simulink model "Assignment_1_3K04"  (R2022b)
settings: Solver=FixedStepAuto  StartTime=0.0  StopTime=1  FixedStep=1e-3  RelTol=1e-3  EnableMultiTasking=on
undefined symbols (not defined in the file): D0, D1, D10, D11, D12, D13, D2, D3, D4, D5, D6, D7, D8, D9, PTA0, PTA1, PTA2, PTB23, PTB9, PTC16, PTC17, PTC2, PTC3, PTC4, PTD0, PTD1, PTD2, PTD3
libraries: frdmk64flib x14
settings Model: ExtModeTrigDuration=5  Creator=Stephen Oh  LastModifiedBy=rebec
settings SolverCC: AlgebraicLoopSolver=TrustRegion
settings OptimizationCC: EnhancedBackFolding=on  PassReuseOutputArgsAs=Individual arguments  ZeroExternalMemoryAtStartup=off  ZeroInternalMemoryAtStartup=off  MaxStackSize=64  OptimizeBlockOrder=speed  DifferentSizesBufferReuse=on  OptimizationCustomize=off  EfficientTunableParamExpr=on
settings DebuggingCC: ParameterTunabilityLossMsg=error  UnconnectedInputMsg=warning  UnconnectedOutputMsg=warning  UnconnectedLineMsg=warning  SFMachineParentedDataDiag=warning
settings HardwareCC: ProdBitPerPointer=32  ProdBitPerSizeT=32  ProdBitPerPtrDiffT=32  ProdLargestAtomicInteger=Long  ProdLargestAtomicFloat=Double  ProdWordSize=32  ProdHWDeviceType=ARM Compatible->ARM Cortex
settings ModelReferenceCC: EnableRefExpFcnMdlSchedulingChecks=on
settings SFSimCC: MATLABDynamicMemAlloc=off
settings RTWCC: Description=Embedded Coder  SystemTargetFile=ert.tlc  HardwareBoard=NXP FRDM-K64F  TLCOptions="-aInlineSetEventsForThisBaseRateFcn=TLC_FALSE -aSuppressMultiTaskScheduler=TLC_FALSE  -aRateBasedStepFcn=0"  TemplateMakefile=ert_default_tmf  Toolchain=GNU Tools for ARM Embedded Processors
settings CodeAppCC: ForceParamTrailComments=on  IgnoreCustomStorageClasses=off  OperatorAnnotations=on  SimulinkDataObjDesc=on  SFDataObjDesc=on  InsertBlockDesc=on

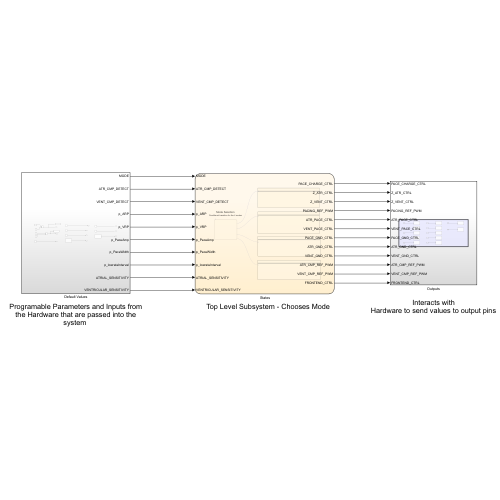
[thumbnail: Simulink's stored preview of the top-level diagram]
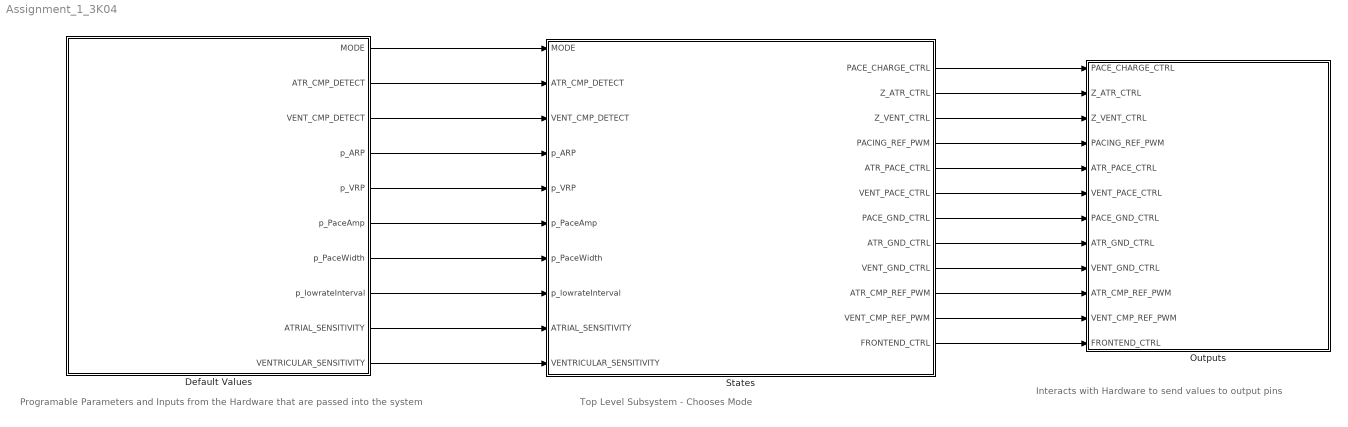
== system Assignment_1_3K04 ==
  note: Programable Parameters and Inputs from the Hardware that are passed into the system
  note: Top Level Subsystem - Chooses Mode
  note: Interacts with
      | Hardware to send values to output pins
  " States" : Stateflow chart  TreatAsAtomicUnit=on
      settings: PortSchema="{\"entries\":[{\"content\":{\"sides\":[{\"content\":{\"connectorIds\":[\"In1\",\"In2\",\"In3\",\"In4\",\"In5\",\"In6\",\"In7\",\"In8\",\"In9\",\"In10\"]},\"type\":\"ConnectorPlacement.EquallySpacedRectSide\",\"uuid\":\"15e03f69-5c25-4f3e-b3fb-d71978e552f4\"},{\"content\":{\"connectorIds\":[\"Out7\",\"Out4\",\"Out5\",\"Out8\",\"Out9\",\"Out3\",\"Out6\",\"Out1\",\"Out2\",\"Out10\",\"Out12\",\"Out11\"],\"side\":\"RIGHT\"},\"type\":\"ConnectorPlacement.EquallySpacedRectSide\",\"uuid\":\"02171bf1-edb1-4b01-9e56-a8642c556ed6\"},{\"content\":{\"connectorIds\":[],\"side\":\"TOP\"},\"type\":\"ConnectorPlacement.EquallySpacedRectSide\",\"uuid\":\"cc6b5506-3435-4740-9e3f-4dfe15d30bff\"}]},\"type\":\"ConnectorPlacement.EquallySpacedConnector\",\"uuid\":\"0ad55da7-1e65-48d0-a0a4-2620ffa94320\"}],\"packageUris\":[\"http://schema.mathworks.com/mf0/Connector/R2020b\"],\"version\":\"1.0\"}"
  Default Values : Subsystem
  Outputs : Subsystem
  wires:
  Default Values/1(MODE) -> " States"/1(MODE)
  Default Values/2(ATR_CMP_DETECT) -> " States"/2(ATR_CMP_DETECT)
  Default Values/3(VENT_CMP_DETECT) -> " States"/3(VENT_CMP_DETECT)
  Default Values/4(p_ARP) -> " States"/4(p_ARP)
  Default Values/5(p_VRP) -> " States"/5(p_VRP)
  Default Values/7(p_PaceWidth) -> " States"/7(p_PaceWidth)
  Default Values/9(ATRIAL_SENSITIVITY) -> " States"/9(ATRIAL_SENSITIVITY)
  Default Values/10(VENTRICULAR_SENSITIVITY) -> " States"/10(VENTRICULAR_SENSITIVITY)
  " States"/7(PACE_CHARGE_CTRL) -> Outputs/1(PACE_CHARGE_CTRL)
  " States"/4(Z_ATR_CTRL) -> Outputs/2(Z_ATR_CTRL)
  " States"/5(Z_VENT_CTRL) -> Outputs/3(Z_VENT_CTRL)
  " States"/8(PACING_REF_PWM) -> Outputs/4(PACING_REF_PWM)
  " States"/9(ATR_PACE_CTRL) -> Outputs/5(ATR_PACE_CTRL)
  " States"/3(VENT_PACE_CTRL) -> Outputs/6(VENT_PACE_CTRL)
  " States"/6(PACE_GND_CTRL) -> Outputs/7(PACE_GND_CTRL)
  " States"/1(ATR_GND_CTRL) -> Outputs/8(ATR_GND_CTRL)
  " States"/2(VENT_GND_CTRL) -> Outputs/9(VENT_GND_CTRL)
  " States"/10(ATR_CMP_REF_PWM) -> Outputs/10(ATR_CMP_REF_PWM)
  " States"/12(VENT_CMP_REF_PWM) -> Outputs/11(VENT_CMP_REF_PWM)
  " States"/11(FRONTEND_CTRL) -> Outputs/12(FRONTEND_CTRL)
  Default Values/8(p_lowrateInterval) -> " States"/8(p_lowrateInterval)
  Default Values/6(p_PaceAmp) -> " States"/6(p_PaceAmp)

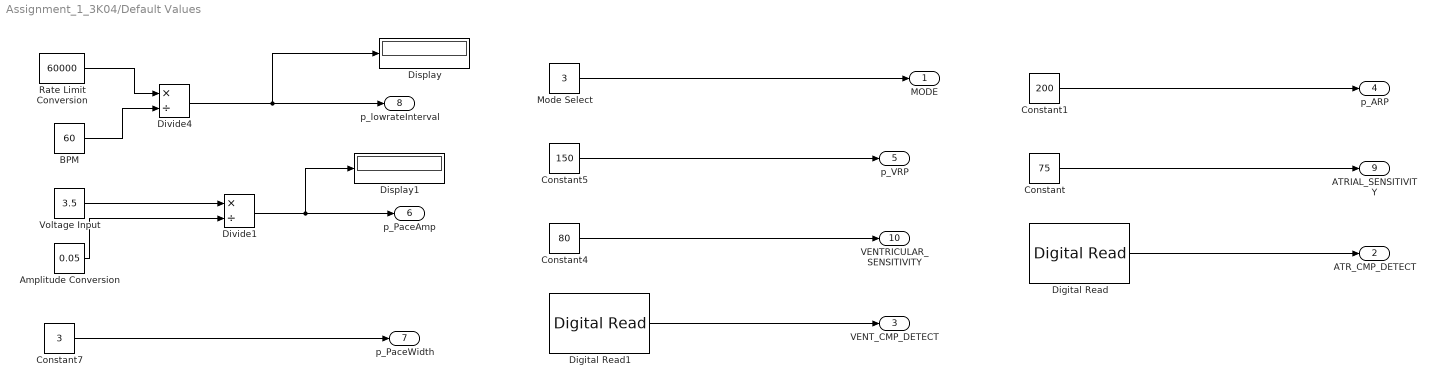
== system Assignment_1_3K04/Default Values ==
  Amplitude Conversion : Constant  Value=0.05
  BPM : Constant  Value=60
  Constant : Constant  Value=75
  Constant1 : Constant  Value=200
  Constant4 : Constant  Value=80
  Constant5 : Constant  Value=150
  Constant7 : Constant  Value=3
  Digital Read : frdmk64flib/Digital Read  Whichpin=PTC16 (D0)  SampleTime=-1
  Digital Read1 : frdmk64flib/Digital Read  Whichpin=PTC17 (D1)  SampleTime=-1
  Display : Display
  Display1 : Display
  Divide1 : Product  Inputs=*/  RndMeth=Nearest
  Divide4 : Product  Inputs=*/  OutDataTypeStr=Inherit: Keep MSB  RndMeth=Nearest
  Mode Select : Constant  Value=3
  Rate Limit Conversion : Constant  Value=60000
  Voltage Input : Constant  Value=3.5
  MODE : Outport
  ATR_CMP_DETECT : Outport  Port=2
  VENT_CMP_DETECT : Outport  Port=3
  p_ARP : Outport  Port=4
  p_VRP : Outport  Port=5
  p_PaceAmp : Outport  Port=6
  p_PaceWidth : Outport  Port=7
  p_lowrateInterval : Outport  Port=8
  ATRIAL_SENSITIVITY : Outport  Port=9
  VENTRICULAR_SENSITIVITY : Outport  Port=10
  wires:
  Mode Select/1 -> MODE/1
  Digital Read/1 -> ATR_CMP_DETECT/1
  Constant7/1 -> p_PaceWidth/1
  Constant1/1 -> p_ARP/1
  Constant/1 -> ATRIAL_SENSITIVITY/1
  Digital Read1/1 -> VENT_CMP_DETECT/1
  Constant4/1 -> VENTRICULAR_SENSITIVITY/1
  Constant5/1 -> p_VRP/1
  Voltage Input/1 -> Divide1/1
  BPM/1 -> Divide4/2
  Divide1/1 -> Display1/1, p_PaceAmp/1
  Amplitude Conversion/1 -> Divide1/2
  Divide4/1 -> p_lowrateInterval/1, Display/1
  Rate Limit Conversion/1 -> Divide4/1

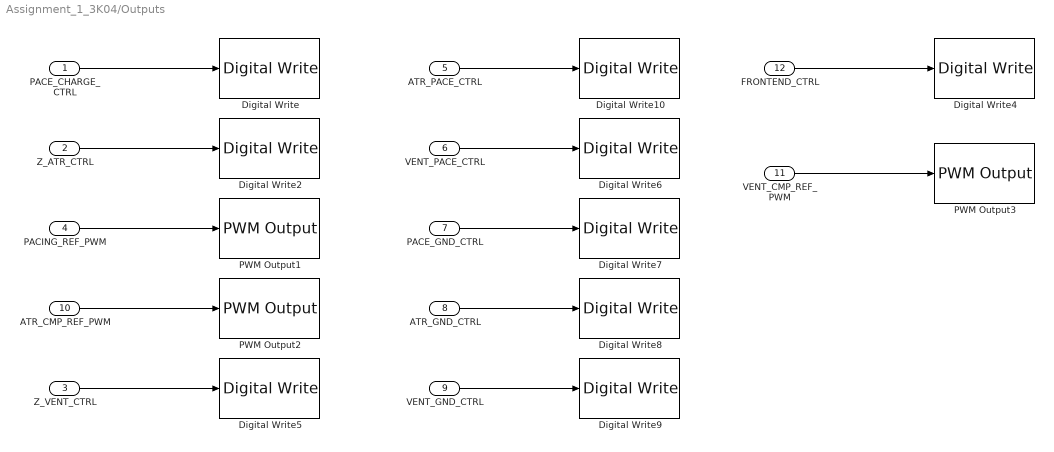
== system Assignment_1_3K04/Outputs ==
  PACE_CHARGE_CTRL : Inport
  Z_ATR_CTRL : Inport  Port=2
  Z_VENT_CTRL : Inport  Port=3
  PACING_REF_PWM : Inport  Port=4
  ATR_PACE_CTRL : Inport  Port=5
  VENT_PACE_CTRL : Inport  Port=6
  PACE_GND_CTRL : Inport  Port=7
  ATR_GND_CTRL : Inport  Port=8
  VENT_GND_CTRL : Inport  Port=9
  ATR_CMP_REF_PWM : Inport  Port=10
  VENT_CMP_REF_PWM : Inport  Port=11
  FRONTEND_CTRL : Inport  Port=12
  Digital Write : frdmk64flib/Digital Write  Whichpin=PTB9 (D2)
  Digital Write10 : frdmk64flib/Digital Write  Whichpin=PTA0 (D8)
  Digital Write2 : frdmk64flib/Digital Write  Whichpin=PTB23 (D4)
  Digital Write4 : frdmk64flib/Digital Write  Whichpin=PTD1 (D13)
  Digital Write5 : frdmk64flib/Digital Write  Whichpin=PTC3 (D7)
  Digital Write6 : frdmk64flib/Digital Write  Whichpin=PTC4 (D9)
  Digital Write7 : frdmk64flib/Digital Write  Whichpin=PTD0 (D10)
  Digital Write8 : frdmk64flib/Digital Write  Whichpin=PTD2 (D11)
  Digital Write9 : frdmk64flib/Digital Write  Whichpin=PTD3 (D12)
  PWM Output1 : frdmk64flib/PWM Output  Whichpin=PTA2 (D5)  InitialFrequency=2000  InitialDutyCycle=0
  PWM Output2 : frdmk64flib/PWM Output  Whichpin=PTC2 (D6)  InitialFrequency=2000  InitialDutyCycle=0
  PWM Output3 : frdmk64flib/PWM Output  Whichpin=PTA1 (D3)  InitialFrequency=2000  InitialDutyCycle=0
  wires:
  ATR_GND_CTRL/1 -> Digital Write8/1
  Z_ATR_CTRL/1 -> Digital Write2/1
  VENT_PACE_CTRL/1 -> Digital Write6/1
  PACING_REF_PWM/1 -> PWM Output1/1
  VENT_GND_CTRL/1 -> Digital Write9/1
  PACE_GND_CTRL/1 -> Digital Write7/1
  FRONTEND_CTRL/1 -> Digital Write4/1
  PACE_CHARGE_CTRL/1 -> Digital Write/1
  Z_VENT_CTRL/1 -> Digital Write5/1
  ATR_CMP_REF_PWM/1 -> PWM Output2/1
  ATR_PACE_CTRL/1 -> Digital Write10/1
  VENT_CMP_REF_PWM/1 -> PWM Output3/1

== stateflow chart Assignment_1_3K04/ States ==
  state AOO [group]
    state Pacing
      entry:
      %charge release of capacitor C22 into C21
      PACE_CHARGE_CTRL = 0;
      PACE_GND_CTRL = 1;
      ATR_PACE_CTRL = 1;
      ATR_GND_CTRL = 0;
      Z_ATR_CTRL = 0;
      Z_VENT_CTRL = 0;
      VENT_GND_CTRL = 0;
      VENT_PACE_CTRL = 0;
    state Discharging
      entry:
      %charging release of capacitor C21 to gnd
      PACE_GND_CTRL = 1;
      VENT_PACE_CTRL = 0;
      Z_ATR_CTRL = 0;
      Z_VENT_CTRL = 0;
      ATR_PACE_CTRL = 0;
      ATR_GND_CTRL = 1;
      VENT_GND_CTRL = 0;
    state Charging
      entry:
      %charging capacitor C22
      ATR_PACE_CTRL = 0;
      VENT_PACE_CTRL = 0;
      PACING_REF_PWM = (p_PaceAmp);
      PACE_CHARGE_CTRL = 1;
    AOO.Pacing -> AOO.Discharging : after(p_PaceWidth, msec)
    AOO.Charging -> AOO.Pacing : after(p_lowrateInterval, msec)
    AOO.Discharging -> AOO.Charging
  note: Mode Selection
  state VOO [group]
    state Charging
      entry:
      %charging capacitor C22
      ATR_PACE_CTRL = 0;
      VENT_PACE_CTRL = 0;
      PACING_REF_PWM = p_PaceAmp;
      PACE_CHARGE_CTRL = 1;
    state Pacing
      entry:
      %charge release of capacitor C22 into C21
      PACE_CHARGE_CTRL = 0;
      PACE_GND_CTRL = 1;
      ATR_PACE_CTRL = 0;
      ATR_GND_CTRL = 0;
      Z_ATR_CTRL = 0;
      Z_VENT_CTRL = 0;
      VENT_GND_CTRL = 0;
      VENT_PACE_CTRL = 1;
    state Discharging
      entry:
      %charging release of capacitor C21 to gnd
      PACE_GND_CTRL = 1;
      VENT_PACE_CTRL = 0;
      Z_ATR_CTRL = 0;
      Z_VENT_CTRL = 0;
      ATR_PACE_CTRL = 0;
      ATR_GND_CTRL = 0;
      VENT_GND_CTRL = 1;
    VOO.Charging -> VOO.Pacing : after(p_lowrateInterval, msec)
    VOO.Pacing -> VOO.Discharging : after(p_PaceWidth, msec)
    VOO.Discharging -> VOO.Charging
  note: Conditional transition for the 4 modes
  state ModeSelect
  state AAI [group]
    state Pacing
      entry:
      %charging release of capacitor C21 to gnd
      PACE_CHARGE_CTRL = 0;
      PACE_GND_CTRL = 1;
      ATR_PACE_CTRL = 1;
      ATR_GND_CTRL = 0;
      Z_ATR_CTRL = 0;
      Z_VENT_CTRL = 0;
      VENT_GND_CTRL = 0;
      VENT_PACE_CTRL = 0;
    state Charging
      entry:
      % turn sensing ON
      FRONTEND_CTRL = 1;
      ATR_CMP_REF_PWM = ATRIAL_SENSITIVITY;
      %charging capacitor C22
      PACING_REF_PWM = p_PaceAmp;
      PACE_CHARGE_CTRL = 1;
      VENT_PACE_CTRL = 0;
      ATR_PACE_CTRL = 0;
    note: Check for intrinsic pulse
    state Discharging
      entry:
      %charging release of capacitor C21 to gnd
      PACE_GND_CTRL = 1;
      VENT_PACE_CTRL = 0;
      ATR_PACE_CTRL = 0;
      Z_ATR_CTRL = 0;
      Z_VENT_CTRL = 0;
      ATR_GND_CTRL = 1;
      VENT_GND_CTRL = 0;
    (junction 150) -> AAI.Charging [order 1] : [ATR_CMP_DETECT == 1]
    AAI.Charging -> (junction 150) : after(p_ARP, msec)
    (junction 150) -> AAI.Pacing [order 2] : after(p_lowrateInterval, msec)
    AAI.Pacing -> AAI.Discharging : after(p_PaceWidth, msec)
    AAI.Discharging -> AAI.Charging
  state VVI [group]
    state Pacing
      entry:
      %charging release of capacitor C21 to gnd
      PACE_CHARGE_CTRL = 0;
      PACE_GND_CTRL = 1;
      ATR_PACE_CTRL = 0;
      ATR_GND_CTRL = 0;
      Z_ATR_CTRL = 0;
      Z_VENT_CTRL = 0;
      VENT_GND_CTRL = 0;
      VENT_PACE_CTRL = 1;
    state Charging
      entry:
      % turn sensing ON
      FRONTEND_CTRL = 1;
      VENT_CMP_REF_PWM = VENTRICULAR_SENSITIVITY;
      %charging capacitor C22
      PACING_REF_PWM = p_PaceAmp;
      PACE_CHARGE_CTRL = 1;
      VENT_PACE_CTRL = 0;
      ATR_PACE_CTRL = 0;
    note: Check for intrinsic pulse
    state Discharging
      entry:
      %charging release of capacitor C21 to gnd
      PACE_GND_CTRL = 1;
      VENT_PACE_CTRL = 0;
      ATR_PACE_CTRL = 0;
      Z_ATR_CTRL = 0;
      Z_VENT_CTRL = 0;
      ATR_GND_CTRL = 0;
      VENT_GND_CTRL = 1;
    (junction 155) -> VVI.Charging [order 1] : [VENT_CMP_DETECT == 1]
    VVI.Charging -> (junction 155) : after(p_VRP, msec)
    (junction 155) -> VVI.Pacing [order 2] : after(p_lowrateInterval, msec)
    VVI.Pacing -> VVI.Discharging : after(p_PaceWidth, msec)
    VVI.Discharging -> VVI.Charging
  ModeSelect -> AOO.Charging [order 1] : [MODE == 0]
  ModeSelect -> VOO.Charging [order 2] : [MODE == 1]
  (default) -> ModeSelect
  ModeSelect -> VVI.Charging [order 4] : [MODE == 3]
  ModeSelect -> AAI.Charging [order 3] : [MODE == 2]
  data: ATR_GND_CTRL output; VENT_GND_CTRL output; VENT_PACE_CTRL output; Z_ATR_CTRL output; Z_VENT_CTRL output; PACE_GND_CTRL output; PACE_CHARGE_CTRL output; PACING_REF_PWM output; ATR_PACE_CTRL output; MODE input; ATR_CMP_REF_PWM output; FRONTEND_CTRL output; VENT_CMP_REF_PWM output; ATR_CMP_DETECT input; VENT_CMP_DETECT input; p_ARP input; p_VRP input; p_PaceAmp input; p_PaceWidth input; p_lowrateInterval input; ATRIAL_SENSITIVITY input; VENTRICULAR_SENSITIVITY input
